simulink model "adder"  (R2016a)
settings: Solver=FixedStepAuto  StartTime=0.0  StopTime=1  FixedStep=.1  RelTol=1e-3
settings Model: Creator=dskaputa  LastModifiedBy=dskaputa
settings HardwareCC: ProdBitPerInt=16  ProdBitPerPointer=16  ProdLargestAtomicFloat=None  ProdWordSize=8  ProdHWDeviceType=Atmel->AVR
settings RTWCC: PackageGeneratedCodeAndArtifacts=on  PackageName=pwm.zip  PostCodeGenCommand=packNGo(buildInfo);  Description=Generic Real-Time Target  GenerateReport=on  RTWVerbose=off  Toolchain=MinGW64 v4.x | gmake (64-bit Windows)  LaunchReport=on
settings CodeAppCC: ForceParamTrailComments=on  OperatorAnnotations=on  MATLABSourceComments=on
settings GRTTargetCC: GeneratePreprocessorConditionals=Use local settings

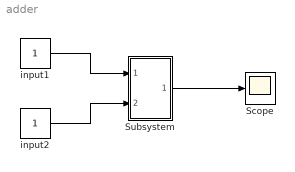
== system adder ==
  Scope : Scope
  Subsystem : Subsystem
  input1 : Constant  OutDataTypeStr=fixdt(1,16,0)
  input2 : Constant  OutDataTypeStr=fixdt(1,16,0)
  wires:
  input1/1 -> Subsystem/1(In1)
  input2/1 -> Subsystem/2(In2)
  Subsystem/1(Out1) -> Scope/1

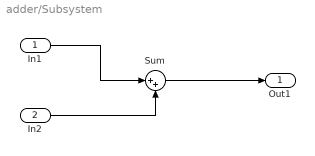
== system adder/Subsystem ==
  In1 : Inport
  In2 : Inport  Port=2
  Sum : Sum  Inputs=|++
  Out1 : Outport
  wires:
  In2/1 -> Sum/2
  Sum/1 -> Out1/1
  In1/1 -> Sum/1
